simulink model "untitled1"  (R2019b)
settings: Solver=VariableStepAuto  StartTime=0.0  StopTime=1  RelTol=1e-3
values from neighbouring files (symbols this model uses):
  d = 23/2    (= 11.5)    [test.m]
  r = 20.5    [test.m]
undefined symbols (not defined in the file or in its folder): a, g, m, zeta_fr
libraries: dspindex x18, dspinverses x1
(part 1 of 2)
settings Model: Creator=arund  LastModifiedBy=arund

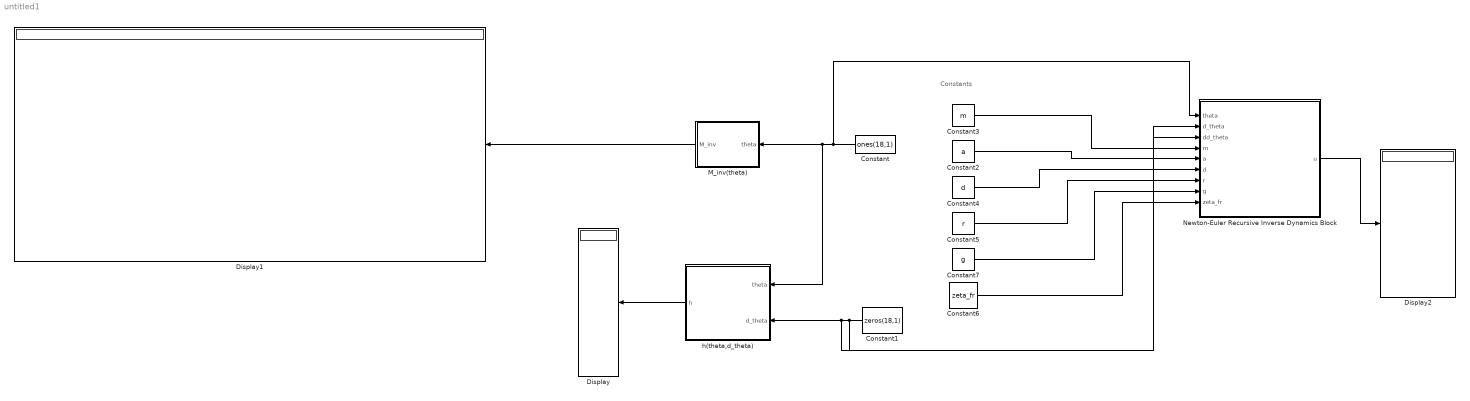
== system untitled1 ==
  note: Constants
  Constant : Constant  Value=ones(18,1)
  Constant1 : Constant  Value=zeros(18,1)
  Constant2 : Constant  Value=a
  Constant3 : Constant  Value=m
  Constant4 : Constant  Value=d
  Constant5 : Constant  Value=r
  Constant6 : Constant  Value=zeta_fr
  Constant7 : Constant  Value=g
  Display : Display
  Display1 : Display
  Display2 : Display
  M_inv(theta) : Subsystem
  Newton-Euler Recursive Inverse Dynamics Block : MATLAB Function  TreatAsAtomicUnit=on
  h(theta,d_theta) : Subsystem
  wires:
  Constant/1 -> Newton-Euler Recursive Inverse Dynamics Block/1(theta), h(theta,d_theta)/1(theta), M_inv(theta)/1(theta)
  Constant1/1 -> Newton-Euler Recursive Inverse Dynamics Block/3(dd_theta), Newton-Euler Recursive Inverse Dynamics Block/2(d_theta), h(theta,d_theta)/2(d_theta)
  h(theta,d_theta)/1(h) -> Display/1
  M_inv(theta)/1(M_inv) -> Display1/1
  Newton-Euler Recursive Inverse Dynamics Block/1(u) -> Display2/1
  Constant7/1 -> Newton-Euler Recursive Inverse Dynamics Block/8(g)
  Constant5/1 -> Newton-Euler Recursive Inverse Dynamics Block/7(r)
  Constant3/1 -> Newton-Euler Recursive Inverse Dynamics Block/4(m)
  Constant4/1 -> Newton-Euler Recursive Inverse Dynamics Block/6(d)
  Constant2/1 -> Newton-Euler Recursive Inverse Dynamics Block/5(a)
  Constant6/1 -> Newton-Euler Recursive Inverse Dynamics Block/9(zeta_fr)

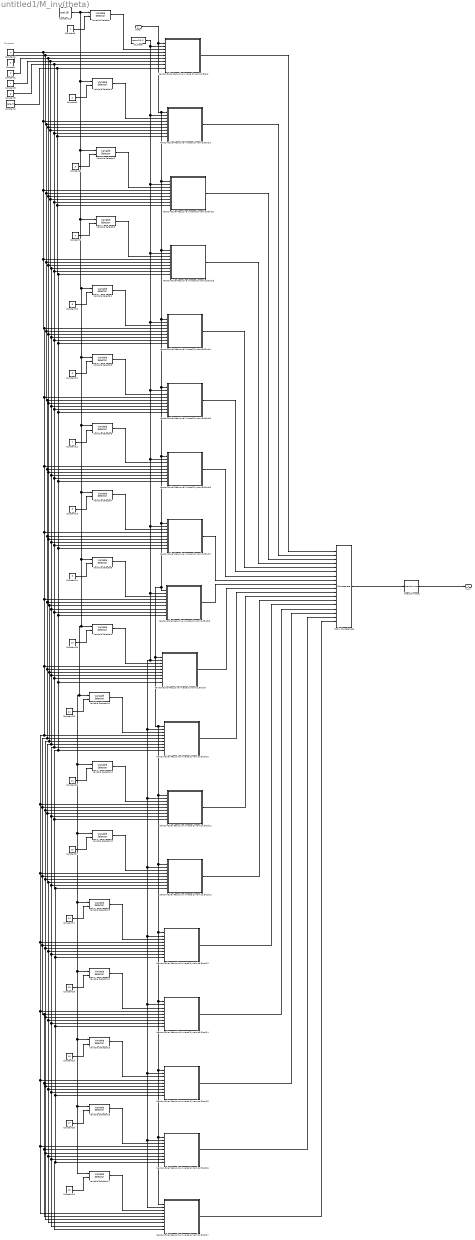
== system untitled1/M_inv(theta) ==
  note: Constants
  theta : Inport
  Constant : Constant  Value=a
  Constant1 : Constant  Value=m
  Constant10 : Constant  Value=5
  Constant11 : Constant  Value=6
  Constant12 : Constant  Value=7
  Constant13 : Constant  Value=8
  Constant14 : Constant  Value=9
  Constant15 : Constant  Value=eye(18)
  Constant17 : Constant  Value=14
  Constant18 : Constant  Value=15
  Constant19 : Constant  Value=16
  Constant2 : Constant  Value=d
  Constant20 : Constant  Value=17
  Constant21 : Constant  Value=18
  Constant26 : Constant  Value=12
  Constant27 : Constant  Value=13
  Constant28 : Constant  Value=10
  Constant29 : Constant  Value=11
  Constant3 : Constant  Value=r
  Constant4 : Constant  Value=zeta_fr
  Constant5 : Constant  Value=g
  Constant6 : Constant  Value=3
  Constant7 : Constant  Value=4
  Constant8 : Constant
  Constant9 : Constant  Value=2
  Matrix Concatenate : Concatenate  NumInputs=18  Mode=Multidimensional array  ConcatenateDimension=2
  Newton-Euler Recursive Inverse Dynamics Block : MATLAB Function  TreatAsAtomicUnit=on
  Newton-Euler Recursive Inverse Dynamics Block1 : MATLAB Function  TreatAsAtomicUnit=on
  Newton-Euler Recursive Inverse Dynamics Block10 : MATLAB Function  TreatAsAtomicUnit=on
  Newton-Euler Recursive Inverse Dynamics Block11 : MATLAB Function  TreatAsAtomicUnit=on
  Newton-Euler Recursive Inverse Dynamics Block12 : MATLAB Function  TreatAsAtomicUnit=on
  Newton-Euler Recursive Inverse Dynamics Block13 : MATLAB Function  TreatAsAtomicUnit=on
  Newton-Euler Recursive Inverse Dynamics Block14 : MATLAB Function  TreatAsAtomicUnit=on
  Newton-Euler Recursive Inverse Dynamics Block15 : MATLAB Function  TreatAsAtomicUnit=on
  Newton-Euler Recursive Inverse Dynamics Block16 : MATLAB Function  TreatAsAtomicUnit=on
  Newton-Euler Recursive Inverse Dynamics Block17 : MATLAB Function  TreatAsAtomicUnit=on
  Newton-Euler Recursive Inverse Dynamics Block2 : MATLAB Function  TreatAsAtomicUnit=on
  Newton-Euler Recursive Inverse Dynamics Block3 : MATLAB Function  TreatAsAtomicUnit=on
  Newton-Euler Recursive Inverse Dynamics Block4 : MATLAB Function  TreatAsAtomicUnit=on
  Newton-Euler Recursive Inverse Dynamics Block5 : MATLAB Function  TreatAsAtomicUnit=on
  Newton-Euler Recursive Inverse Dynamics Block6 : MATLAB Function  TreatAsAtomicUnit=on
  Newton-Euler Recursive Inverse Dynamics Block7 : MATLAB Function  TreatAsAtomicUnit=on
  Newton-Euler Recursive Inverse Dynamics Block8 : MATLAB Function  TreatAsAtomicUnit=on
  Newton-Euler Recursive Inverse Dynamics Block9 : MATLAB Function  TreatAsAtomicUnit=on
  Pseudoinverse : dspinverses/Pseudoinverse  wanterr=off  SimulateUsing=Interpreted execution
      settings: SourceProductName=DSP System Toolbox  SourceProductBaseCode=DS
  Variable Selector{,1..17} (18 alike) : dspindex/Variable Selector  NumInputs=1  rowsOrCols=Columns  IdxMode=Variable  Elements=[1 3]  ZerOneIdxMode=One-based  errmode=Clip Index  FillMode=on  FillValues=0
  dd_theta : Constant  Value=zeros(18,1)
  M_inv : Outport
  wires:
  Newton-Euler Recursive Inverse Dynamics Block/1(u) -> Matrix Concatenate/1
  Variable Selector/1 -> Newton-Euler Recursive Inverse Dynamics Block/3(dd_theta)
  Constant8/1 -> Variable Selector/2
  Variable Selector1/1 -> Newton-Euler Recursive Inverse Dynamics Block1/3(dd_theta)
  Newton-Euler Recursive Inverse Dynamics Block1/1(u) -> Matrix Concatenate/2
  Constant9/1 -> Variable Selector1/2
  Matrix Concatenate/1 -> Pseudoinverse/1
  Constant6/1 -> Variable Selector2/2
  Newton-Euler Recursive Inverse Dynamics Block2/1(u) -> Matrix Concatenate/3
  Variable Selector2/1 -> Newton-Euler Recursive Inverse Dynamics Block2/3(dd_theta)
  Constant7/1 -> Variable Selector3/2
  Newton-Euler Recursive Inverse Dynamics Block3/1(u) -> Matrix Concatenate/4
  Variable Selector3/1 -> Newton-Euler Recursive Inverse Dynamics Block3/3(dd_theta)
  Constant10/1 -> Variable Selector4/2
  Newton-Euler Recursive Inverse Dynamics Block4/1(u) -> Matrix Concatenate/5
  Variable Selector4/1 -> Newton-Euler Recursive Inverse Dynamics Block4/3(dd_theta)
  Constant11/1 -> Variable Selector5/2
  Newton-Euler Recursive Inverse Dynamics Block5/1(u) -> Matrix Concatenate/6
  Variable Selector5/1 -> Newton-Euler Recursive Inverse Dynamics Block5/3(dd_theta)
  Constant12/1 -> Variable Selector6/2
  Newton-Euler Recursive Inverse Dynamics Block6/1(u) -> Matrix Concatenate/7
  Variable Selector6/1 -> Newton-Euler Recursive Inverse Dynamics Block6/3(dd_theta)
  Constant13/1 -> Variable Selector7/2
  Newton-Euler Recursive Inverse Dynamics Block7/1(u) -> Matrix Concatenate/8
  Variable Selector7/1 -> Newton-Euler Recursive Inverse Dynamics Block7/3(dd_theta)
  Constant14/1 -> Variable Selector8/2
  Newton-Euler Recursive Inverse Dynamics Block8/1(u) -> Matrix Concatenate/9
  Variable Selector8/1 -> Newton-Euler Recursive Inverse Dynamics Block8/3(dd_theta)
  Pseudoinverse/1 -> M_inv/1
  Constant3/1 -> Newton-Euler Recursive Inverse Dynamics Block7/7(r), Newton-Euler Recursive Inverse Dynamics Block8/7(r), Newton-Euler Recursive Inverse Dynamics Block9/7(r), Newton-Euler Recursive Inverse Dynamics Block10/7(r), Newton-Euler Recursive Inverse Dynamics Block16/7(r), Newton-Euler Recursive Inverse Dynamics Block17/7(r), Newton-Euler Recursive Inverse Dynamics Block15/7(r), Newton-Euler Recursive Inverse Dynamics Block14/7(r), Newton-Euler Recursive Inverse Dynamics Block13/7(r), Newton-Euler Recursive Inverse Dynamics Block12/7(r), Newton-Euler Recursive Inverse Dynamics Block11/7(r), Newton-Euler Recursive Inverse Dynamics Block6/7(r), Newton-Euler Recursive Inverse Dynamics Block5/7(r), Newton-Euler Recursive Inverse Dynamics Block4/7(r), Newton-Euler Recursive Inverse Dynamics Block3/7(r), Newton-Euler Recursive Inverse Dynamics Block2/7(r), Newton-Euler Recursive Inverse Dynamics Block1/7(r), Newton-Euler Recursive Inverse Dynamics Block/7(r)
  Constant2/1 -> Newton-Euler Recursive Inverse Dynamics Block7/6(d), Newton-Euler Recursive Inverse Dynamics Block8/6(d), Newton-Euler Recursive Inverse Dynamics Block17/6(d), Newton-Euler Recursive Inverse Dynamics Block16/6(d), Newton-Euler Recursive Inverse Dynamics Block15/6(d), Newton-Euler Recursive Inverse Dynamics Block14/6(d), Newton-Euler Recursive Inverse Dynamics Block13/6(d), Newton-Euler Recursive Inverse Dynamics Block12/6(d), Newton-Euler Recursive Inverse Dynamics Block11/6(d), Newton-Euler Recursive Inverse Dynamics Block10/6(d), Newton-Euler Recursive Inverse Dynamics Block9/6(d), Newton-Euler Recursive Inverse Dynamics Block6/6(d), Newton-Euler Recursive Inverse Dynamics Block5/6(d), Newton-Euler Recursive Inverse Dynamics Block4/6(d), Newton-Euler Recursive Inverse Dynamics Block3/6(d), Newton-Euler Recursive Inverse Dynamics Block2/6(d), Newton-Euler Recursive Inverse Dynamics Block1/6(d), Newton-Euler Recursive Inverse Dynamics Block/6(d)
  Variable Selector11/1 -> Newton-Euler Recursive Inverse Dynamics Block11/3(dd_theta)
  Constant26/1 -> Variable Selector11/2
  Newton-Euler Recursive Inverse Dynamics Block10/1(u) -> Matrix Concatenate/11
  Variable Selector14/1 -> Newton-Euler Recursive Inverse Dynamics Block14/3(dd_theta)
  Constant18/1 -> Variable Selector14/2
  Variable Selector17/1 -> Newton-Euler Recursive Inverse Dynamics Block17/3(dd_theta)
  Constant21/1 -> Variable Selector17/2
  Newton-Euler Recursive Inverse Dynamics Block9/1(u) -> Matrix Concatenate/10
  Constant/1 -> Newton-Euler Recursive Inverse Dynamics Block2/5(a), Newton-Euler Recursive Inverse Dynamics Block6/5(a), Newton-Euler Recursive Inverse Dynamics Block7/5(a), Newton-Euler Recursive Inverse Dynamics Block8/5(a), Newton-Euler Recursive Inverse Dynamics Block9/5(a), Newton-Euler Recursive Inverse Dynamics Block11/5(a), Newton-Euler Recursive Inverse Dynamics Block15/5(a), Newton-Euler Recursive Inverse Dynamics Block16/5(a), Newton-Euler Recursive Inverse Dynamics Block17/5(a), Newton-Euler Recursive Inverse Dynamics Block14/5(a), Newton-Euler Recursive Inverse Dynamics Block13/5(a), Newton-Euler Recursive Inverse Dynamics Block12/5(a), Newton-Euler Recursive Inverse Dynamics Block10/5(a), Newton-Euler Recursive Inverse Dynamics Block5/5(a), Newton-Euler Recursive Inverse Dynamics Block4/5(a), Newton-Euler Recursive Inverse Dynamics Block3/5(a), Newton-Euler Recursive Inverse Dynamics Block1/5(a), Newton-Euler Recursive Inverse Dynamics Block/5(a)
  Constant5/1 -> Newton-Euler Recursive Inverse Dynamics Block7/8(g), Newton-Euler Recursive Inverse Dynamics Block8/8(g), Newton-Euler Recursive Inverse Dynamics Block9/8(g), Newton-Euler Recursive Inverse Dynamics Block10/8(g), Newton-Euler Recursive Inverse Dynamics Block17/8(g), Newton-Euler Recursive Inverse Dynamics Block16/8(g), Newton-Euler Recursive Inverse Dynamics Block15/8(g), Newton-Euler Recursive Inverse Dynamics Block14/8(g), Newton-Euler Recursive Inverse Dynamics Block13/8(g), Newton-Euler Recursive Inverse Dynamics Block12/8(g), Newton-Euler Recursive Inverse Dynamics Block11/8(g), Newton-Euler Recursive Inverse Dynamics Block6/8(g), Newton-Euler Recursive Inverse Dynamics Block5/8(g), Newton-Euler Recursive Inverse Dynamics Block4/8(g), Newton-Euler Recursive Inverse Dynamics Block3/8(g), Newton-Euler Recursive Inverse Dynamics Block2/8(g), Newton-Euler Recursive Inverse Dynamics Block1/8(g), Newton-Euler Recursive Inverse Dynamics Block/8(g)
  Constant15/1 -> Variable Selector9/1, Variable Selector10/1, Variable Selector17/1, Variable Selector16/1, Variable Selector15/1, Variable Selector14/1, Variable Selector13/1, Variable Selector12/1, Variable Selector11/1, Variable Selector8/1, Variable Selector7/1, Variable Selector6/1, Variable Selector5/1, Variable Selector4/1, Variable Selector3/1, Variable Selector2/1, Variable Selector1/1, Variable Selector/1
  dd_theta/1 -> Newton-Euler Recursive Inverse Dynamics Block17/2(d_theta), Newton-Euler Recursive Inverse Dynamics Block16/2(d_theta), Newton-Euler Recursive Inverse Dynamics Block15/2(d_theta), Newton-Euler Recursive Inverse Dynamics Block14/2(d_theta), Newton-Euler Recursive Inverse Dynamics Block13/2(d_theta), Newton-Euler Recursive Inverse Dynamics Block12/2(d_theta), Newton-Euler Recursive Inverse Dynamics Block11/2(d_theta), Newton-Euler Recursive Inverse Dynamics Block10/2(d_theta), Newton-Euler Recursive Inverse Dynamics Block9/2(d_theta), Newton-Euler Recursive Inverse Dynamics Block8/2(d_theta), Newton-Euler Recursive Inverse Dynamics Block7/2(d_theta), Newton-Euler Recursive Inverse Dynamics Block6/2(d_theta), Newton-Euler Recursive Inverse Dynamics Block5/2(d_theta), Newton-Euler Recursive Inverse Dynamics Block4/2(d_theta), Newton-Euler Recursive Inverse Dynamics Block3/2(d_theta), Newton-Euler Recursive Inverse Dynamics Block2/2(d_theta), Newton-Euler Recursive Inverse Dynamics Block1/2(d_theta), Newton-Euler Recursive Inverse Dynamics Block/2(d_theta)
  Newton-Euler Recursive Inverse Dynamics Block16/1(u) -> Matrix Concatenate/17
  theta/1 -> Newton-Euler Recursive Inverse Dynamics Block7/1(theta), Newton-Euler Recursive Inverse Dynamics Block16/1(theta), Newton-Euler Recursive Inverse Dynamics Block17/1(theta), Newton-Euler Recursive Inverse Dynamics Block15/1(theta), Newton-Euler Recursive Inverse Dynamics Block14/1(theta), Newton-Euler Recursive Inverse Dynamics Block13/1(theta), Newton-Euler Recursive Inverse Dynamics Block12/1(theta), Newton-Euler Recursive Inverse Dynamics Block11/1(theta), Newton-Euler Recursive Inverse Dynamics Block10/1(theta), Newton-Euler Recursive Inverse Dynamics Block9/1(theta), Newton-Euler Recursive Inverse Dynamics Block8/1(theta), Newton-Euler Recursive Inverse Dynamics Block6/1(theta), Newton-Euler Recursive Inverse Dynamics Block5/1(theta), Newton-Euler Recursive Inverse Dynamics Block4/1(theta), Newton-Euler Recursive Inverse Dynamics Block3/1(theta), Newton-Euler Recursive Inverse Dynamics Block2/1(theta), Newton-Euler Recursive Inverse Dynamics Block1/1(theta), Newton-Euler Recursive Inverse Dynamics Block/1(theta)
  Constant28/1 -> Variable Selector9/2
  Newton-Euler Recursive Inverse Dynamics Block15/1(u) -> Matrix Concatenate/16
  Newton-Euler Recursive Inverse Dynamics Block14/1(u) -> Matrix Concatenate/15
  Variable Selector13/1 -> Newton-Euler Recursive Inverse Dynamics Block13/3(dd_theta)
  Constant17/1 -> Variable Selector13/2
  Constant20/1 -> Variable Selector16/2
  Constant19/1 -> Variable Selector15/2
  Constant29/1 -> Variable Selector10/2
  Variable Selector10/1 -> Newton-Euler Recursive Inverse Dynamics Block10/3(dd_theta)
  Newton-Euler Recursive Inverse Dynamics Block12/1(u) -> Matrix Concatenate/13
  Constant4/1 -> Newton-Euler Recursive Inverse Dynamics Block6/9(zeta_fr), Newton-Euler Recursive Inverse Dynamics Block7/9(zeta_fr), Newton-Euler Recursive Inverse Dynamics Block8/9(zeta_fr), Newton-Euler Recursive Inverse Dynamics Block9/9(zeta_fr), Newton-Euler Recursive Inverse Dynamics Block15/9(zeta_fr), Newton-Euler Recursive Inverse Dynamics Block16/9(zeta_fr), Newton-Euler Recursive Inverse Dynamics Block17/9(zeta_fr), Newton-Euler Recursive Inverse Dynamics Block14/9(zeta_fr), Newton-Euler Recursive Inverse Dynamics Block13/9(zeta_fr), Newton-Euler Recursive Inverse Dynamics Block12/9(zeta_fr), Newton-Euler Recursive Inverse Dynamics Block11/9(zeta_fr), Newton-Euler Recursive Inverse Dynamics Block10/9(zeta_fr), Newton-Euler Recursive Inverse Dynamics Block5/9(zeta_fr), Newton-Euler Recursive Inverse Dynamics Block4/9(zeta_fr), Newton-Euler Recursive Inverse Dynamics Block3/9(zeta_fr), Newton-Euler Recursive Inverse Dynamics Block2/9(zeta_fr), Newton-Euler Recursive Inverse Dynamics Block1/9(zeta_fr), Newton-Euler Recursive Inverse Dynamics Block/9(zeta_fr)
  Newton-Euler Recursive Inverse Dynamics Block11/1(u) -> Matrix Concatenate/12
  Variable Selector9/1 -> Newton-Euler Recursive Inverse Dynamics Block9/3(dd_theta)
  Constant1/1 -> Newton-Euler Recursive Inverse Dynamics Block2/4(m), Newton-Euler Recursive Inverse Dynamics Block7/4(m), Newton-Euler Recursive Inverse Dynamics Block8/4(m), Newton-Euler Recursive Inverse Dynamics Block10/4(m), Newton-Euler Recursive Inverse Dynamics Block11/4(m), Newton-Euler Recursive Inverse Dynamics Block16/4(m), Newton-Euler Recursive Inverse Dynamics Block17/4(m), Newton-Euler Recursive Inverse Dynamics Block15/4(m), Newton-Euler Recursive Inverse Dynamics Block14/4(m), Newton-Euler Recursive Inverse Dynamics Block13/4(m), Newton-Euler Recursive Inverse Dynamics Block12/4(m), Newton-Euler Recursive Inverse Dynamics Block9/4(m), Newton-Euler Recursive Inverse Dynamics Block6/4(m), Newton-Euler Recursive Inverse Dynamics Block5/4(m), Newton-Euler Recursive Inverse Dynamics Block4/4(m), Newton-Euler Recursive Inverse Dynamics Block3/4(m), Newton-Euler Recursive Inverse Dynamics Block1/4(m), Newton-Euler Recursive Inverse Dynamics Block/4(m)
  Constant27/1 -> Variable Selector12/2
  Variable Selector12/1 -> Newton-Euler Recursive Inverse Dynamics Block12/3(dd_theta)
  Newton-Euler Recursive Inverse Dynamics Block13/1(u) -> Matrix Concatenate/14
  Variable Selector15/1 -> Newton-Euler Recursive Inverse Dynamics Block15/3(dd_theta)
  Newton-Euler Recursive Inverse Dynamics Block17/1(u) -> Matrix Concatenate/18
  Variable Selector16/1 -> Newton-Euler Recursive Inverse Dynamics Block16/3(dd_theta)

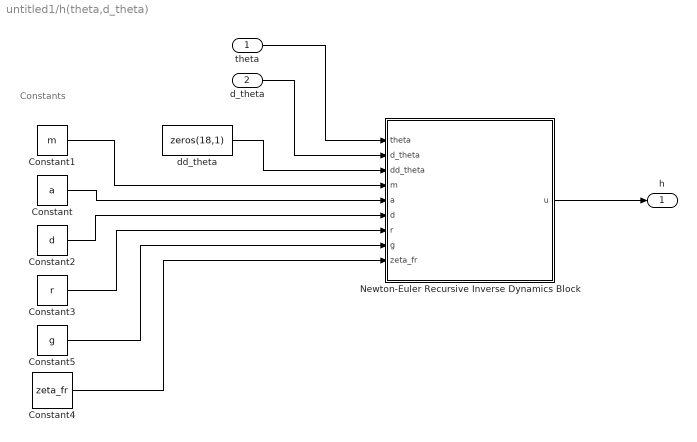
== system untitled1/h(theta,d_theta) ==
  note: Constants
  theta : Inport
  d_theta : Inport  Port=2
  Constant : Constant  Value=a
  Constant1 : Constant  Value=m
  Constant2 : Constant  Value=d
  Constant3 : Constant  Value=r
  Constant4 : Constant  Value=zeta_fr
  Constant5 : Constant  Value=g
  Newton-Euler Recursive Inverse Dynamics Block : MATLAB Function  TreatAsAtomicUnit=on
  dd_theta : Constant  Value=zeros(18,1)
  h : Outport
  wires:
  Newton-Euler Recursive Inverse Dynamics Block/1(u) -> h/1
  d_theta/1 -> Newton-Euler Recursive Inverse Dynamics Block/2(d_theta)
  theta/1 -> Newton-Euler Recursive Inverse Dynamics Block/1(theta)
  Constant2/1 -> Newton-Euler Recursive Inverse Dynamics Block/6(d)
  Constant/1 -> Newton-Euler Recursive Inverse Dynamics Block/5(a)
  Constant3/1 -> Newton-Euler Recursive Inverse Dynamics Block/7(r)
  Constant1/1 -> Newton-Euler Recursive Inverse Dynamics Block/4(m)
  Constant5/1 -> Newton-Euler Recursive Inverse Dynamics Block/8(g)
  Constant4/1 -> Newton-Euler Recursive Inverse Dynamics Block/9(zeta_fr)
  dd_theta/1 -> Newton-Euler Recursive Inverse Dynamics Block/3(dd_theta)

== matlab function untitled1/M_inv(theta)/Newton-Euler Recursive Inverse Dynamics Block1 ==
  data: theta input; u output; d_theta input; dd_theta input; m input; a input; d input; r input; g input; zeta_fr input
%% Neton-Euler Recursive Algorithm for Inverse Dynamics
function u  = fcn(theta, d_theta,dd_theta,m,a,d,r,g,zeta_fr)
%% Parameters
N=9;
P_joint_to_joint=[a+2*d;0;0];
P_link_cm=[-(a/2+d);0;0];
z_0=[0;0;1];
% Create the D-H parameter table
DH_params=zeros(2*N,4);
for i=1:N
    if rem(i,2)==0
        DH_params(2*i-1:2*i,:)=[180+(theta(2*i-1)*180/pi) 90 0 0;...
                                180+(theta(2*i)*180/pi) 0 a 0];
    else
        DH_params(2*i-1:2*i,:)=[theta(2*i-1)*180/pi 90 0 0;...
                                theta(2*i)*180/pi 0 a 0];
    end
end
% Calculate transformation matrix n_A_n+1 (A_wrt_prev) and store in cell
% array
R = cell(2*N,1);
for n=1:2*N
    theta_i=DH_params(n,1);
    alpha_i=DH_params(n,2);
    R{n}=[cosd(theta_i) -sind(theta_i)*cosd(alpha_i) sind(theta_i)*sind(alpha_i);...
       sind(theta_i)  cosd(theta_i)*cosd(alpha_i) -cosd(theta_i)*sind(alpha_i);...
                  0              sind(alpha_i)   cosd(alpha_i) ];
end
% Calculate Inertia tensor
I = cell(N,1);
for i=1:N
    I{i}=[1/12*(m*(a+2*d)^2)+1/4*(m*r^2) 0 0;
                      0 1/12*(m*(a+2*d)^2)+1/4*(m*r^2) 0;
                      0 0 1/4*(m*r^2)];
end
%% Forward recursion
% Initialising the matrices
omega=zeros(3,N);
d_omega=zeros(3,N);
a_joint=zeros(3,N);
a_c=zeros(3,N);
% Initialising prev values
omega_prev=zeros(3,1);
d_omega_prev=zeros(3,1);
a_joint_prev=zeros(3,1);
for n=1:N
    omega(:,n)=(R{2*n-1}*R{2*n})'*(omega_prev + z_0*d_theta(2*n-1)) + ...
               (R{2*n})'*z_0*d_theta(2*n);
    d_omega(:,n)=(R{2*n-1}*R{2*n})'*(d_omega_prev + z_0*dd_theta(2*n-1)+...
                                     cross(omega(:,n),z_0*d_theta(2*n-1))) + ...
                 (R{2*n-1}*R{2*n})'*(cross((z_0*d_theta(2*n-1) + omega_prev),R{2*n-1}*z_0*d_theta(2*n))) + ...
                 (R{2*n})'*(z_0*dd_theta(2*n));
    if n==1
        a_joint(:,n)=[0;0;g];
    else
        a_joint(:,n)=(R{2*n-3}*R{2*n-2})'*a_joint_prev+ ...
                     cross(d_omega_prev,P_joint_to_joint)+...
                     cross(omega_prev,cross(omega_prev,P_joint_to_joint));
    end
    a_c(:,n)=(R{2*n-1}*R{2*n})'*a_joint(:,n)+...
             cross(d_omega(:,n),(P_joint_to_joint+P_link_cm))+...
             cross(omega(:,n),cross(omega(:,n),(P_joint_to_joint+P_link_cm)));
    % Update prev values for next iteration
    omega_prev=omega(:,n);
    d_omega_prev=d_omega(:,n);
    a_joint_prev=a_joint(:,n);
end

%% Backward recursion
% Initialising the matrices
F=zeros(3,N);
tau=zeros(3,N);
% Initialise next values
F_next=zeros(3,1);
tau_next=zeros(3,1);
for n=N:-1:1
   F(:,n) = F_next + m*a_c(:,n);
   tau(:,n) = tau_next - cross(F(:,n),(P_joint_to_joint+P_link_cm)) + ...
              cross(F_next,P_link_cm) + ...
              I{n}*d_omega(:,n)+ cross(omega(:,n),I{n}*omega(:,n));
   % Update next values for next iteration
   F_next=F(:,n);
   tau_next=tau(:,n);
end
%% Computing the output
summed_d_theta=zeros(N,1);
for i=1:N
    summed_d_theta(i)=d_theta(2*i-1)+d_theta(2*i);
end
u=tau'*z_0+(zeta_fr*summed_d_theta);

== matlab function untitled1/M_inv(theta)/Newton-Euler Recursive Inverse Dynamics Block2 ==
  data: theta input; u output; d_theta input; dd_theta input; m input; a input; d input; r input; g input; zeta_fr input
%% Neton-Euler Recursive Algorithm for Inverse Dynamics
function u  = fcn(theta, d_theta,dd_theta,m,a,d,r,g,zeta_fr)
%% Parameters
N=9;
P_joint_to_joint=[a+2*d;0;0];
P_link_cm=[-(a/2+d);0;0];
z_0=[0;0;1];
% Create the D-H parameter table
DH_params=zeros(2*N,4);
for i=1:N
    if rem(i,2)==0
        DH_params(2*i-1:2*i,:)=[180+(theta(2*i-1)*180/pi) 90 0 0;...
                                180+(theta(2*i)*180/pi) 0 a 0];
    else
        DH_params(2*i-1:2*i,:)=[theta(2*i-1)*180/pi 90 0 0;...
                                theta(2*i)*180/pi 0 a 0];
    end
end
% Calculate transformation matrix n_A_n+1 (A_wrt_prev) and store in cell
% array
R = cell(2*N,1);
for n=1:2*N
    theta_i=DH_params(n,1);
    alpha_i=DH_params(n,2);
    R{n}=[cosd(theta_i) -sind(theta_i)*cosd(alpha_i) sind(theta_i)*sind(alpha_i);...
       sind(theta_i)  cosd(theta_i)*cosd(alpha_i) -cosd(theta_i)*sind(alpha_i);...
                  0              sind(alpha_i)   cosd(alpha_i) ];
end
% Calculate Inertia tensor
I = cell(N,1);
for i=1:N
    I{i}=[1/12*(m*(a+2*d)^2)+1/4*(m*r^2) 0 0;
                      0 1/12*(m*(a+2*d)^2)+1/4*(m*r^2) 0;
                      0 0 1/4*(m*r^2)];
end
%% Forward recursion
% Initialising the matrices
omega=zeros(3,N);
d_omega=zeros(3,N);
a_joint=zeros(3,N);
a_c=zeros(3,N);
% Initialising prev values
omega_prev=zeros(3,1);
d_omega_prev=zeros(3,1);
a_joint_prev=zeros(3,1);
for n=1:N
    omega(:,n)=(R{2*n-1}*R{2*n})'*(omega_prev + z_0*d_theta(2*n-1)) + ...
               (R{2*n})'*z_0*d_theta(2*n);
    d_omega(:,n)=(R{2*n-1}*R{2*n})'*(d_omega_prev + z_0*dd_theta(2*n-1)+...
                                     cross(omega(:,n),z_0*d_theta(2*n-1))) + ...
                 (R{2*n-1}*R{2*n})'*(cross((z_0*d_theta(2*n-1) + omega_prev),R{2*n-1}*z_0*d_theta(2*n))) + ...
                 (R{2*n})'*(z_0*dd_theta(2*n));
    if n==1
        a_joint(:,n)=[0;0;g];
    else
        a_joint(:,n)=(R{2*n-3}*R{2*n-2})'*a_joint_prev+ ...
                     cross(d_omega_prev,P_joint_to_joint)+...
                     cross(omega_prev,cross(omega_prev,P_joint_to_joint));
    end
    a_c(:,n)=(R{2*n-1}*R{2*n})'*a_joint(:,n)+...
             cross(d_omega(:,n),(P_joint_to_joint+P_link_cm))+...
             cross(omega(:,n),cross(omega(:,n),(P_joint_to_joint+P_link_cm)));
    % Update prev values for next iteration
    omega_prev=omega(:,n);
    d_omega_prev=d_omega(:,n);
    a_joint_prev=a_joint(:,n);
end

%% Backward recursion
% Initialising the matrices
F=zeros(3,N);
tau=zeros(3,N);
% Initialise next values
F_next=zeros(3,1);
tau_next=zeros(3,1);
for n=N:-1:1
   F(:,n) = F_next + m*a_c(:,n);
   tau(:,n) = tau_next - cross(F(:,n),(P_joint_to_joint+P_link_cm)) + ...
              cross(F_next,P_link_cm) + ...
              I{n}*d_omega(:,n)+ cross(omega(:,n),I{n}*omega(:,n));
   % Update next values for next iteration
   F_next=F(:,n);
   tau_next=tau(:,n);
end
%% Computing the output
summed_d_theta=zeros(N,1);
for i=1:N
    summed_d_theta(i)=d_theta(2*i-1)+d_theta(2*i);
end
u=tau'*z_0+(zeta_fr*summed_d_theta);

== matlab function untitled1/h(theta,d_theta)/Newton-Euler Recursive Inverse Dynamics Block ==
  data: theta input; u output; d_theta input; dd_theta input; m input; a input; d input; r input; g input; zeta_fr input
%% Neton-Euler Recursive Algorithm for Inverse Dynamics
function u  = fcn(theta, d_theta,dd_theta,m,a,d,r,g,zeta_fr)
%% Parameters
N=9;
P_joint_to_joint=[a+2*d;0;0];
P_link_cm=[-(a/2+d);0;0];
z_0=[0;0;1];
% Create the D-H parameter table
DH_params=zeros(2*N,4);
for i=1:N
    if rem(i,2)==0
        DH_params(2*i-1:2*i,:)=[180+(theta(2*i-1)*180/pi) 90 0 0;...
                                180+(theta(2*i)*180/pi) 0 a 0];
    else
        DH_params(2*i-1:2*i,:)=[theta(2*i-1)*180/pi 90 0 0;...
                                theta(2*i)*180/pi 0 a 0];
    end
end
% Calculate transformation matrix n_A_n+1 (A_wrt_prev) and store in cell
% array
R = cell(2*N,1);
for n=1:2*N
    theta_i=DH_params(n,1);
    alpha_i=DH_params(n,2);
    R{n}=[cosd(theta_i) -sind(theta_i)*cosd(alpha_i) sind(theta_i)*sind(alpha_i);...
       sind(theta_i)  cosd(theta_i)*cosd(alpha_i) -cosd(theta_i)*sind(alpha_i);...
                  0              sind(alpha_i)   cosd(alpha_i) ];
end
% Calculate Inertia tensor
I = cell(N,1);
for i=1:N
    I{i}=[1/12*(m*(a+2*d)^2)+1/4*(m*r^2) 0 0;
                      0 1/12*(m*(a+2*d)^2)+1/4*(m*r^2) 0;
                      0 0 1/4*(m*r^2)];
end
%% Forward recursion
% Initialising the matrices
omega=zeros(3,N);
d_omega=zeros(3,N);
a_joint=zeros(3,N);
a_c=zeros(3,N);
% Initialising prev values
omega_prev=zeros(3,1);
d_omega_prev=zeros(3,1);
a_joint_prev=zeros(3,1);
for n=1:N
    omega(:,n)=(R{2*n-1}*R{2*n})'*(omega_prev + z_0*d_theta(2*n-1)) + ...
               (R{2*n})'*z_0*d_theta(2*n);
    d_omega(:,n)=(R{2*n-1}*R{2*n})'*(d_omega_prev + z_0*dd_theta(2*n-1)+...
                                     cross(omega(:,n),z_0*d_theta(2*n-1))) + ...
                 (R{2*n-1}*R{2*n})'*(cross((z_0*d_theta(2*n-1) + omega_prev),R{2*n-1}*z_0*d_theta(2*n))) + ...
                 (R{2*n})'*(z_0*dd_theta(2*n));
    if n==1
        a_joint(:,n)=[0;0;g];
    else
        a_joint(:,n)=(R{2*n-3}*R{2*n-2})'*a_joint_prev+ ...
                     cross(d_omega_prev,P_joint_to_joint)+...
                     cross(omega_prev,cross(omega_prev,P_joint_to_joint));
    end
    a_c(:,n)=(R{2*n-1}*R{2*n})'*a_joint(:,n)+...
             cross(d_omega(:,n),(P_joint_to_joint+P_link_cm))+...
             cross(omega(:,n),cross(omega(:,n),(P_joint_to_joint+P_link_cm)));
    % Update prev values for next iteration
    omega_prev=omega(:,n);
    d_omega_prev=d_omega(:,n);
    a_joint_prev=a_joint(:,n);
end

%% Backward recursion
% Initialising the matrices
F=zeros(3,N);
tau=zeros(3,N);
% Initialise next values
F_next=zeros(3,1);
tau_next=zeros(3,1);
for n=N:-1:1
   F(:,n) = F_next + m*a_c(:,n);
   tau(:,n) = tau_next - cross(F(:,n),(P_joint_to_joint+P_link_cm)) + ...
              cross(F_next,P_link_cm) + ...
              I{n}*d_omega(:,n)+ cross(omega(:,n),I{n}*omega(:,n));
   % Update next values for next iteration
   F_next=F(:,n);
   tau_next=tau(:,n);
end
%% Computing the output
summed_d_theta=zeros(N,1);
for i=1:N
    summed_d_theta(i)=d_theta(2*i-1)+d_theta(2*i);
end
u=tau'*z_0+(zeta_fr*summed_d_theta);

== matlab function untitled1/M_inv(theta)/Newton-Euler Recursive Inverse Dynamics Block10 ==
  data: theta input; u output; d_theta input; dd_theta input; m input; a input; d input; r input; g input; zeta_fr input
%% Neton-Euler Recursive Algorithm for Inverse Dynamics
function u  = fcn(theta, d_theta,dd_theta,m,a,d,r,g,zeta_fr)
%% Parameters
N=9;
P_joint_to_joint=[a+2*d;0;0];
P_link_cm=[-(a/2+d);0;0];
z_0=[0;0;1];
% Create the D-H parameter table
DH_params=zeros(2*N,4);
for i=1:N
    if rem(i,2)==0
        DH_params(2*i-1:2*i,:)=[180+(theta(2*i-1)*180/pi) 90 0 0;...
                                180+(theta(2*i)*180/pi) 0 a 0];
    else
        DH_params(2*i-1:2*i,:)=[theta(2*i-1)*180/pi 90 0 0;...
                                theta(2*i)*180/pi 0 a 0];
    end
end
% Calculate transformation matrix n_A_n+1 (A_wrt_prev) and store in cell
% array
R = cell(2*N,1);
for n=1:2*N
    theta_i=DH_params(n,1);
    alpha_i=DH_params(n,2);
    R{n}=[cosd(theta_i) -sind(theta_i)*cosd(alpha_i) sind(theta_i)*sind(alpha_i);...
       sind(theta_i)  cosd(theta_i)*cosd(alpha_i) -cosd(theta_i)*sind(alpha_i);...
                  0              sind(alpha_i)   cosd(alpha_i) ];
end
% Calculate Inertia tensor
I = cell(N,1);
for i=1:N
    I{i}=[1/12*(m*(a+2*d)^2)+1/4*(m*r^2) 0 0;
                      0 1/12*(m*(a+2*d)^2)+1/4*(m*r^2) 0;
                      0 0 1/4*(m*r^2)];
end
%% Forward recursion
% Initialising the matrices
omega=zeros(3,N);
d_omega=zeros(3,N);
a_joint=zeros(3,N);
a_c=zeros(3,N);
% Initialising prev values
omega_prev=zeros(3,1);
d_omega_prev=zeros(3,1);
a_joint_prev=zeros(3,1);
for n=1:N
    omega(:,n)=(R{2*n-1}*R{2*n})'*(omega_prev + z_0*d_theta(2*n-1)) + ...
               (R{2*n})'*z_0*d_theta(2*n);
    d_omega(:,n)=(R{2*n-1}*R{2*n})'*(d_omega_prev + z_0*dd_theta(2*n-1)+...
                                     cross(omega(:,n),z_0*d_theta(2*n-1))) + ...
                 (R{2*n-1}*R{2*n})'*(cross((z_0*d_theta(2*n-1) + omega_prev),R{2*n-1}*z_0*d_theta(2*n))) + ...
                 (R{2*n})'*(z_0*dd_theta(2*n));
    if n==1
        a_joint(:,n)=[0;0;g];
    else
        a_joint(:,n)=(R{2*n-3}*R{2*n-2})'*a_joint_prev+ ...
                     cross(d_omega_prev,P_joint_to_joint)+...
                     cross(omega_prev,cross(omega_prev,P_joint_to_joint));
    end
    a_c(:,n)=(R{2*n-1}*R{2*n})'*a_joint(:,n)+...
             cross(d_omega(:,n),(P_joint_to_joint+P_link_cm))+...
             cross(omega(:,n),cross(omega(:,n),(P_joint_to_joint+P_link_cm)));
    % Update prev values for next iteration
    omega_prev=omega(:,n);
    d_omega_prev=d_omega(:,n);
    a_joint_prev=a_joint(:,n);
end

%% Backward recursion
% Initialising the matrices
F=zeros(3,N);
tau=zeros(3,N);
% Initialise next values
F_next=zeros(3,1);
tau_next=zeros(3,1);
for n=N:-1:1
   F(:,n) = F_next + m*a_c(:,n);
   tau(:,n) = tau_next - cross(F(:,n),(P_joint_to_joint+P_link_cm)) + ...
              cross(F_next,P_link_cm) + ...
              I{n}*d_omega(:,n)+ cross(omega(:,n),I{n}*omega(:,n));
   % Update next values for next iteration
   F_next=F(:,n);
   tau_next=tau(:,n);
end
%% Computing the output
summed_d_theta=zeros(N,1);
for i=1:N
    summed_d_theta(i)=d_theta(2*i-1)+d_theta(2*i);
end
u=tau'*z_0+(zeta_fr*summed_d_theta);

== matlab function untitled1/M_inv(theta)/Newton-Euler Recursive Inverse Dynamics Block ==
  data: theta input; u output; d_theta input; dd_theta input; m input; a input; d input; r input; g input; zeta_fr input
%% Neton-Euler Recursive Algorithm for Inverse Dynamics
function u  = fcn(theta, d_theta,dd_theta,m,a,d,r,g,zeta_fr)
%% Parameters
N=9;
P_joint_to_joint=[a+2*d;0;0];
P_link_cm=[-(a/2+d);0;0];
z_0=[0;0;1];
% Create the D-H parameter table
DH_params=zeros(2*N,4);
for i=1:N
    if rem(i,2)==0
        DH_params(2*i-1:2*i,:)=[180+(theta(2*i-1)*180/pi) 90 0 0;...
                                180+(theta(2*i)*180/pi) 0 a 0];
    else
        DH_params(2*i-1:2*i,:)=[theta(2*i-1)*180/pi 90 0 0;...
                                theta(2*i)*180/pi 0 a 0];
    end
end
% Calculate transformation matrix n_A_n+1 (A_wrt_prev) and store in cell
% array
R = cell(2*N,1);
for n=1:2*N
    theta_i=DH_params(n,1);
    alpha_i=DH_params(n,2);
    R{n}=[cosd(theta_i) -sind(theta_i)*cosd(alpha_i) sind(theta_i)*sind(alpha_i);...
       sind(theta_i)  cosd(theta_i)*cosd(alpha_i) -cosd(theta_i)*sind(alpha_i);...
                  0              sind(alpha_i)   cosd(alpha_i) ];
end
% Calculate Inertia tensor
I = cell(N,1);
for i=1:N
    I{i}=[1/12*(m*(a+2*d)^2)+1/4*(m*r^2) 0 0;
                      0 1/12*(m*(a+2*d)^2)+1/4*(m*r^2) 0;
                      0 0 1/4*(m*r^2)];
end
%% Forward recursion
% Initialising the matrices
omega=zeros(3,N);
d_omega=zeros(3,N);
a_joint=zeros(3,N);
a_c=zeros(3,N);
% Initialising prev values
omega_prev=zeros(3,1);
d_omega_prev=zeros(3,1);
a_joint_prev=zeros(3,1);
for n=1:N
    omega(:,n)=(R{2*n-1}*R{2*n})'*(omega_prev + z_0*d_theta(2*n-1)) + ...
               (R{2*n})'*z_0*d_theta(2*n);
    d_omega(:,n)=(R{2*n-1}*R{2*n})'*(d_omega_prev + z_0*dd_theta(2*n-1)+...
                                     cross(omega(:,n),z_0*d_theta(2*n-1))) + ...
                 (R{2*n-1}*R{2*n})'*(cross((z_0*d_theta(2*n-1) + omega_prev),R{2*n-1}*z_0*d_theta(2*n))) + ...
                 (R{2*n})'*(z_0*dd_theta(2*n));
    if n==1
        a_joint(:,n)=[0;0;g];
    else
        a_joint(:,n)=(R{2*n-3}*R{2*n-2})'*a_joint_prev+ ...
                     cross(d_omega_prev,P_joint_to_joint)+...
                     cross(omega_prev,cross(omega_prev,P_joint_to_joint));
    end
    a_c(:,n)=(R{2*n-1}*R{2*n})'*a_joint(:,n)+...
             cross(d_omega(:,n),(P_joint_to_joint+P_link_cm))+...
             cross(omega(:,n),cross(omega(:,n),(P_joint_to_joint+P_link_cm)));
    % Update prev values for next iteration
    omega_prev=omega(:,n);
    d_omega_prev=d_omega(:,n);
    a_joint_prev=a_joint(:,n);
end

%% Backward recursion
% Initialising the matrices
F=zeros(3,N);
tau=zeros(3,N);
% Initialise next values
F_next=zeros(3,1);
tau_next=zeros(3,1);
for n=N:-1:1
   F(:,n) = F_next + m*a_c(:,n);
   tau(:,n) = tau_next - cross(F(:,n),(P_joint_to_joint+P_link_cm)) + ...
              cross(F_next,P_link_cm) + ...
              I{n}*d_omega(:,n)+ cross(omega(:,n),I{n}*omega(:,n));
   % Update next values for next iteration
   F_next=F(:,n);
   tau_next=tau(:,n);
end
%% Computing the output
summed_d_theta=zeros(N,1);
for i=1:N
    summed_d_theta(i)=d_theta(2*i-1)+d_theta(2*i);
end
u=tau'*z_0+(zeta_fr*summed_d_theta);

== matlab function untitled1/Newton-Euler Recursive Inverse Dynamics Block ==
  data: theta input; u output; d_theta input; dd_theta input; m input; a input; d input; r input; g input; zeta_fr input
%% Neton-Euler Recursive Algorithm for Inverse Dynamics
function u  = fcn(theta, d_theta,dd_theta,m,a,d,r,g,zeta_fr)
%% Parameters
N=9;
P_joint_to_joint=[a+2*d;0;0];
P_link_cm=[-(a/2+d);0;0];
z_0=[0;0;1];
% Create the D-H parameter table
DH_params=zeros(2*N,4);
for i=1:N
    if rem(i,2)==0
        DH_params(2*i-1:2*i,:)=[180+(theta(2*i-1)*180/pi) 90 0 0;...
                                180+(theta(2*i)*180/pi) 0 a 0];
    else
        DH_params(2*i-1:2*i,:)=[theta(2*i-1)*180/pi 90 0 0;...
                                theta(2*i)*180/pi 0 a 0];
    end
end
% Calculate transformation matrix n_A_n+1 (A_wrt_prev) and store in cell
% array
R = cell(2*N,1);
for n=1:2*N
    theta_i=DH_params(n,1);
    alpha_i=DH_params(n,2);
    R{n}=[cosd(theta_i) -sind(theta_i)*cosd(alpha_i) sind(theta_i)*sind(alpha_i);...
       sind(theta_i)  cosd(theta_i)*cosd(alpha_i) -cosd(theta_i)*sind(alpha_i);...
                  0              sind(alpha_i)   cosd(alpha_i) ];
end
% Calculate Inertia tensor
I = cell(N,1);
for i=1:N
    I{i}=[1/12*(m*(a+2*d)^2)+1/4*(m*r^2) 0 0;
                      0 1/12*(m*(a+2*d)^2)+1/4*(m*r^2) 0;
                      0 0 1/4*(m*r^2)];
end
%% Forward recursion
% Initialising the matrices
omega=zeros(3,N);
d_omega=zeros(3,N);
a_joint=zeros(3,N);
a_c=zeros(3,N);
% Initialising prev values
omega_prev=zeros(3,1);
d_omega_prev=zeros(3,1);
a_joint_prev=zeros(3,1);
for n=1:N
    omega(:,n)=(R{2*n-1}*R{2*n})'*(omega_prev + z_0*d_theta(2*n-1)) + ...
               (R{2*n})'*z_0*d_theta(2*n);
    d_omega(:,n)=(R{2*n-1}*R{2*n})'*(d_omega_prev + z_0*dd_theta(2*n-1)+...
                                     cross(omega(:,n),z_0*d_theta(2*n-1))) + ...
                 (R{2*n-1}*R{2*n})'*(cross((z_0*d_theta(2*n-1) + omega_prev),R{2*n-1}*z_0*d_theta(2*n))) + ...
                 (R{2*n})'*(z_0*dd_theta(2*n));
    if n==1
        a_joint(:,n)=[0;0;g];
    else
        a_joint(:,n)=(R{2*n-3}*R{2*n-2})'*a_joint_prev+ ...
                     cross(d_omega_prev,P_joint_to_joint)+...
                     cross(omega_prev,cross(omega_prev,P_joint_to_joint));
    end
    a_c(:,n)=(R{2*n-1}*R{2*n})'*a_joint(:,n)+...
             cross(d_omega(:,n),(P_joint_to_joint+P_link_cm))+...
             cross(omega(:,n),cross(omega(:,n),(P_joint_to_joint+P_link_cm)));
    % Update prev values for next iteration
    omega_prev=omega(:,n);
    d_omega_prev=d_omega(:,n);
    a_joint_prev=a_joint(:,n);
end

%% Backward recursion
% Initialising the matrices
F=zeros(3,N);
tau=zeros(3,N);
% Initialise next values
F_next=zeros(3,1);
tau_next=zeros(3,1);
for n=N:-1:1
   F(:,n) = F_next + m*a_c(:,n);
   tau(:,n) = tau_next - cross(F(:,n),(P_joint_to_joint+P_link_cm)) + ...
              cross(F_next,P_link_cm) + ...
              I{n}*d_omega(:,n)+ cross(omega(:,n),I{n}*omega(:,n));
   % Update next values for next iteration
   F_next=F(:,n);
   tau_next=tau(:,n);
end
%% Computing the output
summed_d_theta=zeros(N,1);
for i=1:N
    summed_d_theta(i)=d_theta(2*i-1)+d_theta(2*i);
end
u=tau'*z_0+(zeta_fr*summed_d_theta);

== matlab function untitled1/M_inv(theta)/Newton-Euler Recursive Inverse Dynamics Block3 ==
  data: theta input; u output; d_theta input; dd_theta input; m input; a input; d input; r input; g input; zeta_fr input
%% Neton-Euler Recursive Algorithm for Inverse Dynamics
function u  = fcn(theta, d_theta,dd_theta,m,a,d,r,g,zeta_fr)
%% Parameters
N=9;
P_joint_to_joint=[a+2*d;0;0];
P_link_cm=[-(a/2+d);0;0];
z_0=[0;0;1];
% Create the D-H parameter table
DH_params=zeros(2*N,4);
for i=1:N
    if rem(i,2)==0
        DH_params(2*i-1:2*i,:)=[180+(theta(2*i-1)*180/pi) 90 0 0;...
                                180+(theta(2*i)*180/pi) 0 a 0];
    else
        DH_params(2*i-1:2*i,:)=[theta(2*i-1)*180/pi 90 0 0;...
                                theta(2*i)*180/pi 0 a 0];
    end
end
% Calculate transformation matrix n_A_n+1 (A_wrt_prev) and store in cell
% array
R = cell(2*N,1);
for n=1:2*N
    theta_i=DH_params(n,1);
    alpha_i=DH_params(n,2);
    R{n}=[cosd(theta_i) -sind(theta_i)*cosd(alpha_i) sind(theta_i)*sind(alpha_i);...
       sind(theta_i)  cosd(theta_i)*cosd(alpha_i) -cosd(theta_i)*sind(alpha_i);...
                  0              sind(alpha_i)   cosd(alpha_i) ];
end
% Calculate Inertia tensor
I = cell(N,1);
for i=1:N
    I{i}=[1/12*(m*(a+2*d)^2)+1/4*(m*r^2) 0 0;
                      0 1/12*(m*(a+2*d)^2)+1/4*(m*r^2) 0;
                      0 0 1/4*(m*r^2)];
end
%% Forward recursion
% Initialising the matrices
omega=zeros(3,N);
d_omega=zeros(3,N);
a_joint=zeros(3,N);
a_c=zeros(3,N);
% Initialising prev values
omega_prev=zeros(3,1);
d_omega_prev=zeros(3,1);
a_joint_prev=zeros(3,1);
for n=1:N
    omega(:,n)=(R{2*n-1}*R{2*n})'*(omega_prev + z_0*d_theta(2*n-1)) + ...
               (R{2*n})'*z_0*d_theta(2*n);
    d_omega(:,n)=(R{2*n-1}*R{2*n})'*(d_omega_prev + z_0*dd_theta(2*n-1)+...
                                     cross(omega(:,n),z_0*d_theta(2*n-1))) + ...
                 (R{2*n-1}*R{2*n})'*(cross((z_0*d_theta(2*n-1) + omega_prev),R{2*n-1}*z_0*d_theta(2*n))) + ...
                 (R{2*n})'*(z_0*dd_theta(2*n));
    if n==1
        a_joint(:,n)=[0;0;g];
    else
        a_joint(:,n)=(R{2*n-3}*R{2*n-2})'*a_joint_prev+ ...
                     cross(d_omega_prev,P_joint_to_joint)+...
                     cross(omega_prev,cross(omega_prev,P_joint_to_joint));
    end
    a_c(:,n)=(R{2*n-1}*R{2*n})'*a_joint(:,n)+...
             cross(d_omega(:,n),(P_joint_to_joint+P_link_cm))+...
             cross(omega(:,n),cross(omega(:,n),(P_joint_to_joint+P_link_cm)));
    % Update prev values for next iteration
    omega_prev=omega(:,n);
    d_omega_prev=d_omega(:,n);
    a_joint_prev=a_joint(:,n);
end

%% Backward recursion
% Initialising the matrices
F=zeros(3,N);
tau=zeros(3,N);
% Initialise next values
F_next=zeros(3,1);
tau_next=zeros(3,1);
for n=N:-1:1
   F(:,n) = F_next + m*a_c(:,n);
   tau(:,n) = tau_next - cross(F(:,n),(P_joint_to_joint+P_link_cm)) + ...
              cross(F_next,P_link_cm) + ...
              I{n}*d_omega(:,n)+ cross(omega(:,n),I{n}*omega(:,n));
   % Update next values for next iteration
   F_next=F(:,n);
   tau_next=tau(:,n);
end
%% Computing the output
summed_d_theta=zeros(N,1);
for i=1:N
    summed_d_theta(i)=d_theta(2*i-1)+d_theta(2*i);
end
u=tau'*z_0+(zeta_fr*summed_d_theta);

== matlab function untitled1/M_inv(theta)/Newton-Euler Recursive Inverse Dynamics Block4 ==
  data: theta input; u output; d_theta input; dd_theta input; m input; a input; d input; r input; g input; zeta_fr input
%% Neton-Euler Recursive Algorithm for Inverse Dynamics
function u  = fcn(theta, d_theta,dd_theta,m,a,d,r,g,zeta_fr)
%% Parameters
N=9;
P_joint_to_joint=[a+2*d;0;0];
P_link_cm=[-(a/2+d);0;0];
z_0=[0;0;1];
% Create the D-H parameter table
DH_params=zeros(2*N,4);
for i=1:N
    if rem(i,2)==0
        DH_params(2*i-1:2*i,:)=[180+(theta(2*i-1)*180/pi) 90 0 0;...
                                180+(theta(2*i)*180/pi) 0 a 0];
    else
        DH_params(2*i-1:2*i,:)=[theta(2*i-1)*180/pi 90 0 0;...
                                theta(2*i)*180/pi 0 a 0];
    end
end
% Calculate transformation matrix n_A_n+1 (A_wrt_prev) and store in cell
% array
R = cell(2*N,1);
for n=1:2*N
    theta_i=DH_params(n,1);
    alpha_i=DH_params(n,2);
    R{n}=[cosd(theta_i) -sind(theta_i)*cosd(alpha_i) sind(theta_i)*sind(alpha_i);...
       sind(theta_i)  cosd(theta_i)*cosd(alpha_i) -cosd(theta_i)*sind(alpha_i);...
                  0              sind(alpha_i)   cosd(alpha_i) ];
end
% Calculate Inertia tensor
I = cell(N,1);
for i=1:N
    I{i}=[1/12*(m*(a+2*d)^2)+1/4*(m*r^2) 0 0;
                      0 1/12*(m*(a+2*d)^2)+1/4*(m*r^2) 0;
                      0 0 1/4*(m*r^2)];
end
%% Forward recursion
% Initialising the matrices
omega=zeros(3,N);
d_omega=zeros(3,N);
a_joint=zeros(3,N);
a_c=zeros(3,N);
% Initialising prev values
omega_prev=zeros(3,1);
d_omega_prev=zeros(3,1);
a_joint_prev=zeros(3,1);
for n=1:N
    omega(:,n)=(R{2*n-1}*R{2*n})'*(omega_prev + z_0*d_theta(2*n-1)) + ...
               (R{2*n})'*z_0*d_theta(2*n);
    d_omega(:,n)=(R{2*n-1}*R{2*n})'*(d_omega_prev + z_0*dd_theta(2*n-1)+...
                                     cross(omega(:,n),z_0*d_theta(2*n-1))) + ...
                 (R{2*n-1}*R{2*n})'*(cross((z_0*d_theta(2*n-1) + omega_prev),R{2*n-1}*z_0*d_theta(2*n))) + ...
                 (R{2*n})'*(z_0*dd_theta(2*n));
    if n==1
        a_joint(:,n)=[0;0;g];
    else
        a_joint(:,n)=(R{2*n-3}*R{2*n-2})'*a_joint_prev+ ...
                     cross(d_omega_prev,P_joint_to_joint)+...
                     cross(omega_prev,cross(omega_prev,P_joint_to_joint));
    end
    a_c(:,n)=(R{2*n-1}*R{2*n})'*a_joint(:,n)+...
             cross(d_omega(:,n),(P_joint_to_joint+P_link_cm))+...
             cross(omega(:,n),cross(omega(:,n),(P_joint_to_joint+P_link_cm)));
    % Update prev values for next iteration
    omega_prev=omega(:,n);
    d_omega_prev=d_omega(:,n);
    a_joint_prev=a_joint(:,n);
end

%% Backward recursion
% Initialising the matrices
F=zeros(3,N);
tau=zeros(3,N);
% Initialise next values
F_next=zeros(3,1);
tau_next=zeros(3,1);
for n=N:-1:1
   F(:,n) = F_next + m*a_c(:,n);
   tau(:,n) = tau_next - cross(F(:,n),(P_joint_to_joint+P_link_cm)) + ...
              cross(F_next,P_link_cm) + ...
              I{n}*d_omega(:,n)+ cross(omega(:,n),I{n}*omega(:,n));
   % Update next values for next iteration
   F_next=F(:,n);
   tau_next=tau(:,n);
end
%% Computing the output
summed_d_theta=zeros(N,1);
for i=1:N
    summed_d_theta(i)=d_theta(2*i-1)+d_theta(2*i);
end
u=tau'*z_0+(zeta_fr*summed_d_theta);

== matlab function untitled1/M_inv(theta)/Newton-Euler Recursive Inverse Dynamics Block5 ==
  data: theta input; u output; d_theta input; dd_theta input; m input; a input; d input; r input; g input; zeta_fr input
%% Neton-Euler Recursive Algorithm for Inverse Dynamics
function u  = fcn(theta, d_theta,dd_theta,m,a,d,r,g,zeta_fr)
%% Parameters
N=9;
P_joint_to_joint=[a+2*d;0;0];
P_link_cm=[-(a/2+d);0;0];
z_0=[0;0;1];
% Create the D-H parameter table
DH_params=zeros(2*N,4);
for i=1:N
    if rem(i,2)==0
        DH_params(2*i-1:2*i,:)=[180+(theta(2*i-1)*180/pi) 90 0 0;...
                                180+(theta(2*i)*180/pi) 0 a 0];
    else
        DH_params(2*i-1:2*i,:)=[theta(2*i-1)*180/pi 90 0 0;...
                                theta(2*i)*180/pi 0 a 0];
    end
end
% Calculate transformation matrix n_A_n+1 (A_wrt_prev) and store in cell
% array
R = cell(2*N,1);
for n=1:2*N
    theta_i=DH_params(n,1);
    alpha_i=DH_params(n,2);
    R{n}=[cosd(theta_i) -sind(theta_i)*cosd(alpha_i) sind(theta_i)*sind(alpha_i);...
       sind(theta_i)  cosd(theta_i)*cosd(alpha_i) -cosd(theta_i)*sind(alpha_i);...
                  0              sind(alpha_i)   cosd(alpha_i) ];
end
% Calculate Inertia tensor
I = cell(N,1);
for i=1:N
    I{i}=[1/12*(m*(a+2*d)^2)+1/4*(m*r^2) 0 0;
                      0 1/12*(m*(a+2*d)^2)+1/4*(m*r^2) 0;
                      0 0 1/4*(m*r^2)];
end
%% Forward recursion
% Initialising the matrices
omega=zeros(3,N);
d_omega=zeros(3,N);
a_joint=zeros(3,N);
a_c=zeros(3,N);
% Initialising prev values
omega_prev=zeros(3,1);
d_omega_prev=zeros(3,1);
a_joint_prev=zeros(3,1);
for n=1:N
    omega(:,n)=(R{2*n-1}*R{2*n})'*(omega_prev + z_0*d_theta(2*n-1)) + ...
               (R{2*n})'*z_0*d_theta(2*n);
    d_omega(:,n)=(R{2*n-1}*R{2*n})'*(d_omega_prev + z_0*dd_theta(2*n-1)+...
                                     cross(omega(:,n),z_0*d_theta(2*n-1))) + ...
                 (R{2*n-1}*R{2*n})'*(cross((z_0*d_theta(2*n-1) + omega_prev),R{2*n-1}*z_0*d_theta(2*n))) + ...
                 (R{2*n})'*(z_0*dd_theta(2*n));
    if n==1
        a_joint(:,n)=[0;0;g];
    else
        a_joint(:,n)=(R{2*n-3}*R{2*n-2})'*a_joint_prev+ ...
                     cross(d_omega_prev,P_joint_to_joint)+...
                     cross(omega_prev,cross(omega_prev,P_joint_to_joint));
    end
    a_c(:,n)=(R{2*n-1}*R{2*n})'*a_joint(:,n)+...
             cross(d_omega(:,n),(P_joint_to_joint+P_link_cm))+...
             cross(omega(:,n),cross(omega(:,n),(P_joint_to_joint+P_link_cm)));
    % Update prev values for next iteration
    omega_prev=omega(:,n);
    d_omega_prev=d_omega(:,n);
    a_joint_prev=a_joint(:,n);
end

%% Backward recursion
% Initialising the matrices
F=zeros(3,N);
tau=zeros(3,N);
% Initialise next values
F_next=zeros(3,1);
tau_next=zeros(3,1);
for n=N:-1:1
   F(:,n) = F_next + m*a_c(:,n);
   tau(:,n) = tau_next - cross(F(:,n),(P_joint_to_joint+P_link_cm)) + ...
              cross(F_next,P_link_cm) + ...
              I{n}*d_omega(:,n)+ cross(omega(:,n),I{n}*omega(:,n));
   % Update next values for next iteration
   F_next=F(:,n);
   tau_next=tau(:,n);
end
%% Computing the output
summed_d_theta=zeros(N,1);
for i=1:N
    summed_d_theta(i)=d_theta(2*i-1)+d_theta(2*i);
end
u=tau'*z_0+(zeta_fr*summed_d_theta);
